simulink model "trial_2"  (R2021b)
settings: Solver=VariableStepAuto  StartTime=0.0  StopTime=inf  RelTol=1e-3
values from neighbouring files (symbols this model uses):
  L = 1.96    [setUpPurePursuitCurveLowVel.m]
  ld = 0.5    [setUpPurePursuitCurveLowVel.m]
libraries: robotlib x11, simulink x2, robotalgslib x1
settings Model: Creator=Asus ROG  LastModifiedBy=Asus ROG

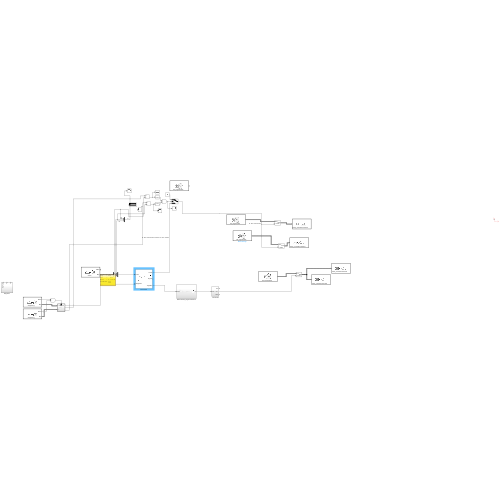
[thumbnail: Simulink's stored preview of the top-level diagram]
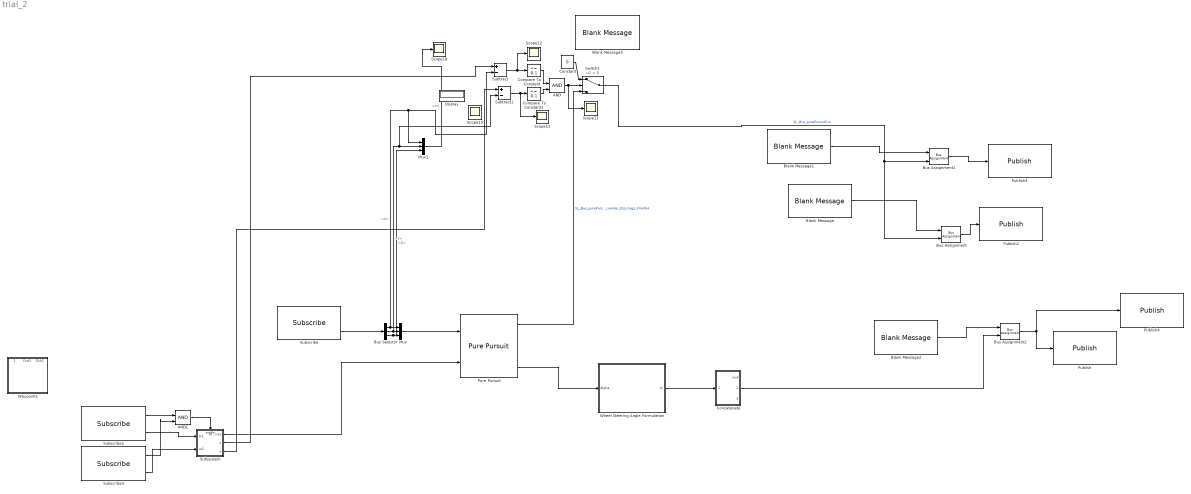
== system trial_2 ==
  AND : Logic  IconShape=distinctive  AllPortsSameDT=off  OutDataTypeStr=boolean
  AND1 : Logic  IconShape=distinctive  AllPortsSameDT=off  OutDataTypeStr=boolean
  Blank Message{,1..3} (4 alike) : robotlib/Blank Message  messageClass=Message  entityType=std_msgs/Float64  messageType=std_msgs/Float64  SampleTime=inf  legacyBusStruct=off
  Bus Assignment : BusAssignment  AssignedSignals=Data
  Bus Assignment1 : BusAssignment  AssignedSignals=Data
  Bus Assignment2 : BusAssignment  AssignedSignals=Data
  Bus Selector : BusSelector  OutputSignals=Pose.Pose.Position.X,Pose.Pose.Position.Y,Twist.Twist.Linear.Z
  Compare To Constant : simulink/Logic and Bit Operations/Compare To Constant  relop=<=  const=0.1  OutDataTypeStr=boolean
  Compare To Constant1 : simulink/Logic and Bit Operations/Compare To Constant  relop=<=  const=0.1  OutDataTypeStr=boolean
  Concatenate : Subsystem
  Constant : Constant  Value=0
  Display : Display
  Mux : Mux  Inputs=3
  Mux1 : Mux  Inputs=3
  Publish : robotlib/Publish  topicSource=Select from ROS network  topic=/follower_zamboni/left_steering_hinge_position_controller/command  messageType=std_msgs/Float64  legacyBusStruct=off  messageQueueLength=1
  Publish2 : robotlib/Publish  topicSource=Select from ROS network  topic=/follower_zamboni/left_rear_wheel_velocity_controller/command  messageType=std_msgs/Float64  legacyBusStruct=off  messageQueueLength=1
  Publish3 : robotlib/Publish  topicSource=Select from ROS network  topic=/follower_zamboni/right_rear_wheel_velocity_controller/command  messageType=std_msgs/Float64  legacyBusStruct=off  messageQueueLength=1
  Publish4 : robotlib/Publish  topicSource=Select from ROS network  topic=/follower_zamboni/right_steering_hinge_position_controller/command  messageType=std_msgs/Float64  legacyBusStruct=off  messageQueueLength=1
  Pure Pursuit : robotalgslib/Pure Pursuit  DesiredLinearVelocity=2  MaxAngularVelocity=5  LookaheadDistance=ld  TargetDirPort=on  SimulateUsing=Code generation
  Scope{10..13,15} (5 alike) : Scope
  Subscribe : robotlib/Subscribe  topicSource=Select from ROS network  topic=/odom  messageType=nav_msgs/Odometry  SampleTime=-1  legacyBusStruct=off  messageQueueLength=1
  Subscribe2 : robotlib/Subscribe  topicSource=Select from ROS network  topic=/waypoints_x  messageType=std_msgs/Float64  SampleTime=-1  legacyBusStruct=off  messageQueueLength=1
  Subscribe3 : robotlib/Subscribe  topicSource=Select from ROS network  topic=/waypoints_y  messageType=std_msgs/Float64  SampleTime=-1  legacyBusStruct=off  messageQueueLength=1
  Subsystem : Subsystem
  Subtract : Sum  Inputs=+-
  Subtract1 : Sum  Inputs=+-
  Switch1 : Switch  Criteria=u2 > Threshold
  Waypoints : Subsystem
      settings: PortSchema="{\"entries\":[{\"content\":{\"sides\":[{\"content\":{\"connectorIds\":[]},\"type\":\"ConnectorPlacement.EquallySpacedRectSide\",\"uuid\":\"1aef6d80-e8a9-4fb7-8510-b2c9f7879556\"},{\"content\":{\"connectorIds\":[],\"side\":\"RIGHT\"},\"type\":\"ConnectorPlacement.EquallySpacedRectSide\",\"uuid\":\"ca868ae5-f684-48a7-9a57-a6a9932b3d7c\"},{\"content\":{\"connectorIds\":[\"Out1\",\"Out2\",\"Out3\"],\"side\":\"TOP\"},\"type\":\"ConnectorPlacement.EquallySpacedRectSide\",\"uuid\":\"53e5d444-9164-44c4-9d78-994de9471315\"}]},\"type\":\"ConnectorPlacement.EquallySpacedConnector\",\"uuid\":\"edcfc3a4-0663-40f8-8137-2b87bcbb479d\"}],\"packageUris\":[\"http://schema.mathworks.com/mf0/Connector/R2020b\"],\"version\":\"1.0\"}"
  Wheel Steering Angle Formulation : Subsystem
  wires:
  Subscribe/2 -> Bus Selector/1
  Mux/1 -> Pure Pursuit/1
  Subsystem/1(WayPoints) -> Pure Pursuit/2
  Pure Pursuit/3 -> Wheel Steering Angle Formulation/1(alpha)
  Wheel Steering Angle Formulation/1(Al) -> Concatenate/1(delta)
  Bus Assignment2/1 -> Publish/1, Publish4/1
  Blank Message2/1 -> Bus Assignment2/1
  Concatenate/2(AnF1) -> Bus Assignment2/2
  Blank Message1/1 -> Bus Assignment1/1
  Blank Message/1 -> Bus Assignment/1
  Switch1/1 -> Bus Assignment/2, Bus Assignment1/2  "SL_Bus_purePursuitCur"
  Bus Assignment/1 -> Publish2/1
  Bus Assignment1/1 -> Publish3/1
  Bus Selector/3 -> Mux1/3, Mux/3  "<Z>"
  Pure Pursuit/1 -> Switch1/3  "SL_Bus_purePursuitCurveLowVel_std_msgs_Float64"
  Compare To Constant1/1 -> AND/2
  AND/1 -> Scope11/1, Switch1/2
  Constant/1 -> Switch1/1
  Subtract1/1 -> Scope13/1, Compare To Constant1/1
  Compare To Constant/1 -> AND/1
  Mux1/1 -> Scope10/1  "<Y>"
  ? -> ?  "<Y>"
  Bus Selector/1 -> Subtract/2, Mux1/1, Mux/1  "<X>"
  Bus Selector/2 -> Subtract1/2, Mux1/2, Mux/2  "<Y>"
  Subtract/1 -> Scope12/1, Compare To Constant/1
  Subsystem/2(x) -> Subtract/1
  Subsystem/3(y) -> Subtract1/1
  Subscribe3/2 -> Subsystem/2(In2)
  Subscribe2/2 -> Subsystem/1(In1)
  Subscribe3/1 -> AND1/2
  AND1/1 -> Subsystem/Enable
  Subscribe2/1 -> AND1/1

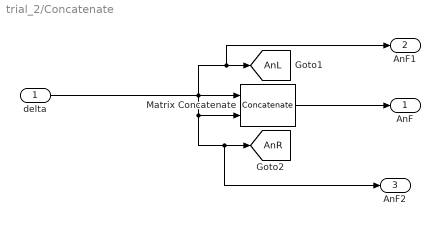
== system trial_2/Concatenate ==
  delta : Inport
  Matrix Concatenate : Concatenate
  AnF : Outport  VectorParamsAs1DForOutWhenUnconnected=off
  AnF1 : Outport  Port=2  VectorParamsAs1DForOutWhenUnconnected=off
  AnF2 : Outport  Port=3  VectorParamsAs1DForOutWhenUnconnected=off
  tag scope: AnL=global, AnR=global
  wires:
  Matrix Concatenate/1 -> AnF/1
  delta/1 -> AnF1/1, [AnL], AnF2/1, [AnR], Matrix Concatenate/2, Matrix Concatenate/1

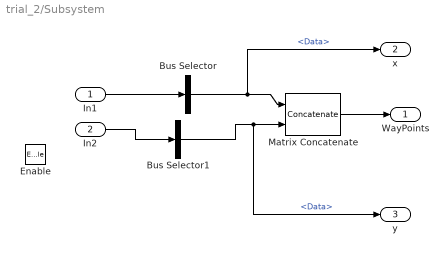
== system trial_2/Subsystem ==
  In1 : Inport
  In2 : Inport  Port=2
  Enable : EnablePort
  Bus Selector : BusSelector  OutputSignals=Data
  Bus Selector1 : BusSelector  OutputSignals=Data
  Matrix Concatenate : Concatenate  Mode=Multidimensional array  ConcatenateDimension=2
  WayPoints : Outport
  x : Outport  Port=2
  y : Outport  Port=3
  wires:
  In1/1 -> Bus Selector/1
  Matrix Concatenate/1 -> WayPoints/1
  In2/1 -> Bus Selector1/1
  Bus Selector/1 -> x/1, Matrix Concatenate/1  "<Data>"
  Bus Selector1/1 -> y/1, Matrix Concatenate/2  "<Data>"

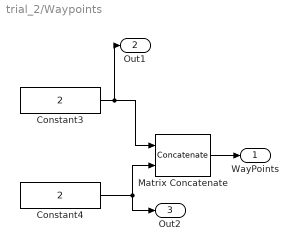
== system trial_2/Waypoints ==
  Constant3 : Constant  Value=2  SampleTime=0.1
  Constant4 : Constant  Value=2  SampleTime=0.1
  Matrix Concatenate : Concatenate  Mode=Multidimensional array  ConcatenateDimension=2
  WayPoints : Outport
  Out1 : Outport  Port=2
  Out2 : Outport  Port=3
  wires:
  Constant4/1 -> Out2/1, Matrix Concatenate/2
  Constant3/1 -> Out1/1, Matrix Concatenate/1
  Matrix Concatenate/1 -> WayPoints/1

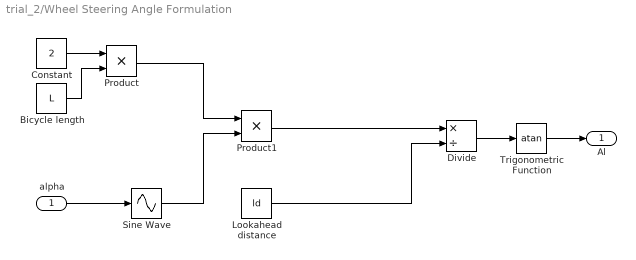
== system trial_2/Wheel Steering Angle Formulation ==
  alpha : Inport
  Bicycle length : Constant  Value=L
  Constant : Constant  Value=2
  Divide : Product  Inputs=*/
  Lookahead distance : Constant  Value=ld
  Product : Product
  Product1 : Product
  Sine Wave : Sin  TimeSource=Use external signal  SampleTime=0
  Trigonometric Function : Trigonometry  Operator=atan
  Al : Outport
  wires:
  Sine Wave/1 -> Product1/2
  Bicycle length/1 -> Product/2
  Constant/1 -> Product/1
  Product1/1 -> Divide/1
  Product/1 -> Product1/1
  Divide/1 -> Trigonometric Function/1
  Trigonometric Function/1 -> Al/1
  alpha/1 -> Sine Wave/1
  Lookahead distance/1 -> Divide/2
